simulink subsystem "Desat_Supervisor"  (R2025a)
settings: Solver=VariableStepAuto  StartTime=0.0  StopTime=10.0  RelTol=1e-3
undefined symbols (not defined in the file): cfg
settings Model: Creator=Jackt  LastModifiedBy=Jackt

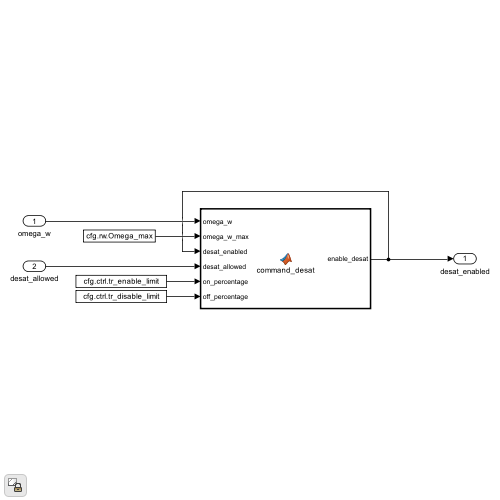
[thumbnail: Simulink's stored preview of the top-level diagram]
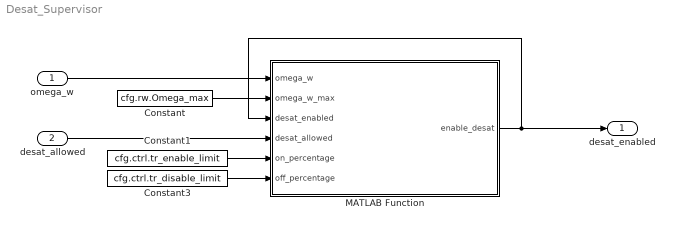
== system Desat_Supervisor ==
  omega_w : Inport
  desat_allowed : Inport  Port=2
  Constant : Constant  Value=cfg.rw.Omega_max
  Constant1 : Constant  Value=cfg.ctrl.tr_enable_limit
  Constant3 : Constant  Value=cfg.ctrl.tr_disable_limit
  MATLAB Function : MATLAB Function  TreatAsAtomicUnit=on
  desat_enabled : Outport
  wires:
  omega_w/1 -> MATLAB Function/1(omega_w)
  desat_allowed/1 -> MATLAB Function/4(desat_allowed)
  MATLAB Function/1(enable_desat) -> MATLAB Function/3(desat_enabled), desat_enabled/1
  Constant/1 -> MATLAB Function/2(omega_w_max)
  Constant1/1 -> MATLAB Function/5(on_percentage)
  Constant3/1 -> MATLAB Function/6(off_percentage)

== matlab function Desat_Supervisor/MATLAB Function ==
  data: omega_w input; omega_w_max input; desat_enabled input; desat_allowed input; enable_desat output; on_percentage input; off_percentage input
function enable_desat = command_desat(omega_w, omega_w_max, desat_enabled, desat_allowed, on_percentage, off_percentage)
%COMMAND_DESAT  Reaction wheel desaturation mode latch (hysteresis).
%
% This function implements a simple hysteresis-based enable/disable latch:
% - If desaturation is not allowed, force OFF.
% - If currently OFF, turn ON when any wheel exceeds the ON threshold.
% - If currently ON, turn OFF only when all wheels are below the OFF threshold.
% - Otherwise hold the current state.
%
% Inputs
%   omega_w        [3x1] wheel speeds (rad/s), signed
%   omega_w_max    scalar max allowable wheel speed magnitude (rad/s)
%   desat_enabled  scalar logical, current desat mode state (latched)
%   desat_allowed  scalar logical, global allow flag from sim settings
%   on_percentage  scalar fraction (0-1), e.g. 0.80
%   off_percentage scalar fraction (0-1), e.g. 0.50
%
% Output
%   enable_desat   scalar logical, next desat mode state

    % ---- Safety / settings gate ----
    % If the sim settings say desaturation is not allowed, force it off.
    if ~desat_allowed
        enable_desat = false;
        return
    end

    % ---- Thresholds (magnitudes) ----
    on_thresh  = omega_w_max * on_percentage;
    off_thresh = omega_w_max * off_percentage;

    % Turn ON if any wheel speed magnitude exceeds the ON threshold
    turn_on  = any(abs(omega_w) > on_thresh);

    % Turn OFF only if all wheel speed magnitudes are below the OFF threshold
    turn_off = all(abs(omega_w) < off_thresh);

    % ---- Hysteresis latch ----
    if ~desat_enabled && turn_on
        enable_desat = true;
    elseif desat_enabled && turn_off
        enable_desat = false;
    else
        enable_desat = logical(desat_enabled);
    end
end
